simulink model "zero_to_hero_sect6"  (R2023a)
settings: Solver=VariableStepAuto  StartTime=0.0  StopTime=sim_time  MaxStep=0.01  RelTol=1e-3
values from neighbouring files (symbols this model uses):
  OCV = table2array(data(:, 2))    [battery_assgn.m]
  R_charge = table2array(data(:, 3))    [battery_assgn.m]
  R_discharge = table2array(data(:, 4))    [battery_assgn.m]
  SOC = table2array(data(:, 1))    [battery_assgn.m]
undefined symbols (not defined in the file or in its folder): C_n, I
settings Model: Creator=fycce  LastModifiedBy=fycce

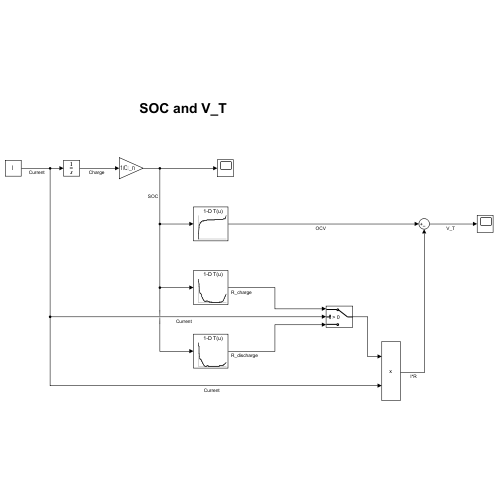
[thumbnail: Simulink's stored preview of the top-level diagram]
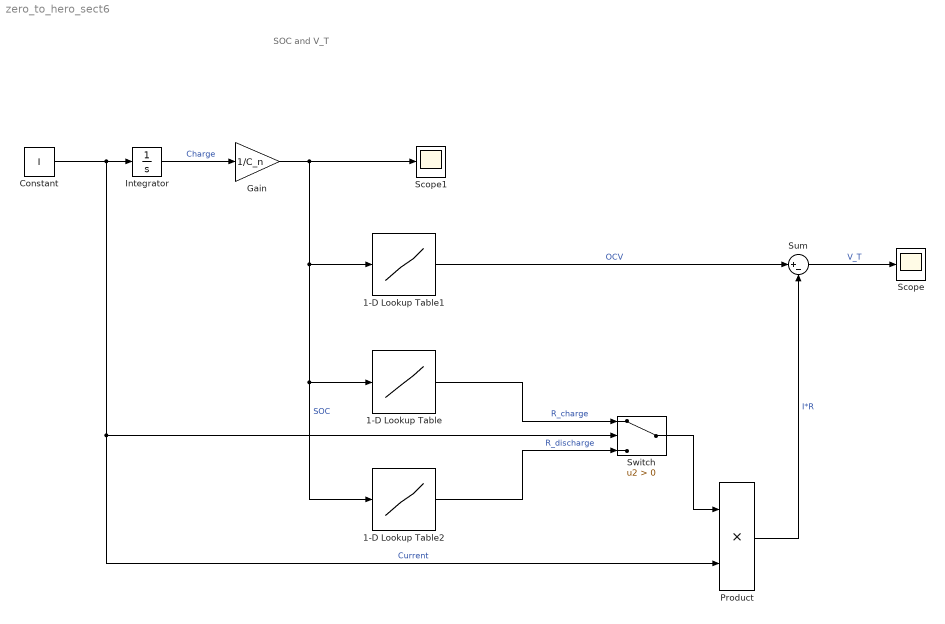
== system zero_to_hero_sect6 ==
  note: SOC and V_T
  1-D Lookup Table : Lookup_n-D  NumberOfTableDimensions=1  BreakpointsForDimension1=SOC  Table=R_charge  InternalRulePriority=Speed  RndMeth=Simplest
  1-D Lookup Table1 : Lookup_n-D  NumberOfTableDimensions=1  BreakpointsForDimension1=SOC  Table=OCV  InternalRulePriority=Speed  RndMeth=Simplest
  1-D Lookup Table2 : Lookup_n-D  NumberOfTableDimensions=1  BreakpointsForDimension1=SOC  Table=R_discharge  InternalRulePriority=Speed  RndMeth=Simplest
  Constant : Constant  Value=I
  Gain : Gain  Gain=1/C_n
  Integrator : Integrator
  Product : Product
  Scope : Scope
  Scope1 : Scope
  Sum : Sum  Inputs=|+-
  Switch : Switch  Criteria=u2 > Threshold  SaturateOnIntegerOverflow=off  InputSameDT=off
  wires:
  Constant/1 -> Integrator/1, Product/2, Switch/2  "Current"
  Integrator/1 -> Gain/1  "Charge"
  Gain/1 -> Scope1/1, 1-D Lookup Table2/1, 1-D Lookup Table/1, 1-D Lookup Table1/1  "SOC"
  1-D Lookup Table1/1 -> Sum/1  "OCV"
  Product/1 -> Sum/2  "I*R"
  Sum/1 -> Scope/1  "V_T"
  Switch/1 -> Product/1
  1-D Lookup Table/1 -> Switch/1  "R_charge"
  1-D Lookup Table2/1 -> Switch/3  "R_discharge"
